simulink model "MCity_cs_withAEBSBlock"  (R2017a)
settings: Solver=ode5  StartTime=0.0  StopTime=3.95  FixedStep=1/200  RelTol=1e-3
PreLoadFcn:
  | check_NUTS_defined;
  | 
  | assignin('base',['model_closed_' bdroot],false);
InitFcn:
  | PreScanExperimentInitFcn(bdroot)
StopFcn:
  | PreScanExperimentStopFcn(bdroot)
model workspace (MAT data in the model file):
  mbox_table : struct (value not decoded)
  model_closed = 0
  sim_status = 0
values from neighbouring files (symbols this model uses):
  d_offset = -18.15    [monocityTestLeftTurn.mat]    (also in simulation_leftTurn_PreScan.m = dl/vl*vh - 43 + R)
undefined symbols (not defined in the file or in its folder): DiscIntNeverNeededParam, warningInitialVelocity, x0
libraries: simulink x78, PreScanSimulinkLibrary x14, simulink_extras x10, PreScanUsefulBlocks x4
(part 2 of 12)

== system MCity_cs_withAEBSBlock/STATE_BMW_Z3_1 ==
  State : Inport  SampleTime=TimeStep
  Acceleration : Subsystem  mask(ToSensorWorld){PortName=Acceleration_BMW_Z3_1, PortIndex=21, PortWidth=3, TimeStep=1/200}
      mask prompts: PortName "Port Name [-]"; PortIndex "Index [-]"; PortWidth "Port Dimensions [-]"; TimeStep "Upload Period [s]"
      mask help: Sends signal(s) from Simulink to the Sensor World
      mask Help:
      | Sends signal(s) from Simulink to the Sensor World.
      | 
      | - Port Name [-]: specifies the name of the output terminal of the Simulink block.
      | - Index [-]: specifies the start position in the output vector sent to the Sensor World
      | - Port dimensions [-]: specifies the width (number of scalars) of the output port
      | - Upload period [s]: specifies the upload period (in seconds) of the port.
      mask Display: port_label('input', 1, PortName)
  Demux : Demux  Outputs=5
  Position : Subsystem  mask(ToSensorWorld){PortName=Position_BMW_Z3_1, PortIndex=15, PortWidth=3, TimeStep=1/200}
      mask prompts: PortName "Port Name [-]"; PortIndex "Index [-]"; PortWidth "Port Dimensions [-]"; TimeStep "Upload Period [s]"
      mask help: Sends signal(s) from Simulink to the Sensor World
      mask Help:
      | Sends signal(s) from Simulink to the Sensor World.
      | 
      | - Port Name [-]: specifies the name of the output terminal of the Simulink block.
      | - Index [-]: specifies the start position in the output vector sent to the Sensor World
      | - Port dimensions [-]: specifies the width (number of scalars) of the output port
      | - Upload period [s]: specifies the upload period (in seconds) of the port.
      mask Display: port_label('input', 1, PortName)
  RPY : Subsystem  mask(ToSensorWorld){PortName=RPY_BMW_Z3_1, PortIndex=24, PortWidth=3, TimeStep=1/200}
      mask prompts: PortName "Port Name [-]"; PortIndex "Index [-]"; PortWidth "Port Dimensions [-]"; TimeStep "Upload Period [s]"
      mask help: Sends signal(s) from Simulink to the Sensor World
      mask Help:
      | Sends signal(s) from Simulink to the Sensor World.
      | 
      | - Port Name [-]: specifies the name of the output terminal of the Simulink block.
      | - Index [-]: specifies the start position in the output vector sent to the Sensor World
      | - Port dimensions [-]: specifies the width (number of scalars) of the output port
      | - Upload period [s]: specifies the upload period (in seconds) of the port.
      mask Display: port_label('input', 1, PortName)
  Velocity : Subsystem  mask(ToSensorWorld){PortName=Velocity_BMW_Z3_1, PortIndex=18, PortWidth=3, TimeStep=1/200}
      mask prompts: PortName "Port Name [-]"; PortIndex "Index [-]"; PortWidth "Port Dimensions [-]"; TimeStep "Upload Period [s]"
      mask help: Sends signal(s) from Simulink to the Sensor World
      mask Help:
      | Sends signal(s) from Simulink to the Sensor World.
      | 
      | - Port Name [-]: specifies the name of the output terminal of the Simulink block.
      | - Index [-]: specifies the start position in the output vector sent to the Sensor World
      | - Port dimensions [-]: specifies the width (number of scalars) of the output port
      | - Upload period [s]: specifies the upload period (in seconds) of the port.
      mask Display: port_label('input', 1, PortName)
  iniBODYAngles wrtVEH [rad] : Constant  Value=[Roll0 Pitch0 0]  SampleTime=TimeStep
  iniVEHAngles wrtGLOB [rad] : Constant  Value=[0 0 Yaw0]  SampleTime=TimeStep
  iniVEHposition wrtGLOB [m] : Constant  Value=[x0 y0+d_offset z0]  SampleTime=TimeStep
  state2FullState : PreScanSimulinkLibrary/state2FullState  SystemSampleTime=-1
  velRPY : Subsystem  mask(ToSensorWorld){PortName=velRPY_BMW_Z3_1, PortIndex=27, PortWidth=3, TimeStep=1/200}
      mask prompts: PortName "Port Name [-]"; PortIndex "Index [-]"; PortWidth "Port Dimensions [-]"; TimeStep "Upload Period [s]"
      mask help: Sends signal(s) from Simulink to the Sensor World
      mask Help:
      | Sends signal(s) from Simulink to the Sensor World.
      | 
      | - Port Name [-]: specifies the name of the output terminal of the Simulink block.
      | - Index [-]: specifies the start position in the output vector sent to the Sensor World
      | - Port dimensions [-]: specifies the width (number of scalars) of the output port
      | - Upload period [s]: specifies the upload period (in seconds) of the port.
      mask Display: port_label('input', 1, PortName)
  wires:
  Demux/5 -> velRPY/1(Y)
  Demux/4 -> RPY/1(Y)
  Demux/3 -> Acceleration/1(Y)
  Demux/2 -> Velocity/1(Y)
  Demux/1 -> Position/1(Y)
  State/1 -> state2FullState/1
  state2FullState/1 -> Demux/1
  iniVEHposition wrtGLOB [m]/1 -> state2FullState/2
  iniBODYAngles wrtVEH [rad]/1 -> state2FullState/3
  iniVEHAngles wrtGLOB [rad]/1 -> state2FullState/4

== system MCity_cs_withAEBSBlock/SetActuators ==
  Bus Creator : BusCreator  Inputs=1
  Data Store Read : DataStoreRead  DataStoreName=SimCoreActuators  SampleTime=TimeStep
  SendActuators : M-S-Function  FunctionName=SendActuatorsBlock  Parameters=TimeStep NrOfActuators
  dummy : Outport
  tag scope: SimCoreInfo=global
  wires:
  Bus Creator/1 -> [SimCoreInfo]  "SimCore"
  SendActuators/2 -> Bus Creator/1  "ComputationTime[s]"
  SendActuators/1 -> dummy/1
  Data Store Read/1 -> SendActuators/1

== system MCity_cs_withAEBSBlock/SimCoreInfo ==
  Bus Selector : BusSelector  OutputSignals=ComputationTime[s]
  Time : Scope
  wires:
  Bus Selector/1 -> Time/1  "<ComputationTime[s]>"
  [SimCoreInfo] -> Bus Selector/1

== system MCity_cs_withAEBSBlock/TrafficLightDoubleUS_1 ==
  Ground_1 : Ground
  "Traffic_Light On/Off " : Subsystem
  VISUCasingLights_1_Mux : Subsystem  Tag=MuxCasingLights  mask(PreScan Mux Block:){}
      settings: DeleteFcn=PreScanBlockDeleteFcn;
  VISUCasingLights_2_Mux : Subsystem  Tag=MuxCasingLights  mask(PreScan Mux Block:){}
      settings: DeleteFcn=PreScanBlockDeleteFcn;
  VISUCasingLights_1_TrafficLightDoubleUS_1 : Outport  Tag=VisuCasingLights_1Outport  SampleTime=1/200
  VISUCasingLights_2_TrafficLightDoubleUS_1 : Outport  Tag=VisuCasingLights_2Outport  Port=2  SampleTime=1/200
  wires:
  VISUCasingLights_2_Mux/1(CasingLights) -> VISUCasingLights_2_TrafficLightDoubleUS_1/1
  VISUCasingLights_1_Mux/1(CasingLights) -> VISUCasingLights_1_TrafficLightDoubleUS_1/1
  "Traffic_Light On/Off "/3(Green) -> VISUCasingLights_1_Mux/3(Green [-]), VISUCasingLights_2_Mux/3(Green [-])
  "Traffic_Light On/Off "/2(Orange) -> VISUCasingLights_1_Mux/2(Orange [-]), VISUCasingLights_2_Mux/2(Orange [-])
  "Traffic_Light On/Off "/1(Red) -> VISUCasingLights_1_Mux/1(Red [-]), VISUCasingLights_2_Mux/1(Red [-])

== system MCity_cs_withAEBSBlock/TrafficLightDoubleUS_10 ==
  Perpendicular : Subsystem
  VISUCasingLights_1_Mux : Subsystem  Tag=MuxCasingLights  mask(PreScan Mux Block:){}
      settings: DeleteFcn=PreScanBlockDeleteFcn;
  VISUCasingLights_2_Mux : Subsystem  Tag=MuxCasingLights  mask(PreScan Mux Block:){}
      settings: DeleteFcn=PreScanBlockDeleteFcn;
  VISUCasingLights_1_TrafficLightDoubleUS_10 : Outport  Tag=VisuCasingLights_1Outport  SampleTime=1/200
  VISUCasingLights_2_TrafficLightDoubleUS_10 : Outport  Tag=VisuCasingLights_2Outport  Port=2  SampleTime=1/200
  wires:
  VISUCasingLights_2_Mux/1(CasingLights) -> VISUCasingLights_2_TrafficLightDoubleUS_10/1
  VISUCasingLights_1_Mux/1(CasingLights) -> VISUCasingLights_1_TrafficLightDoubleUS_10/1
  Perpendicular/3(Green) -> VISUCasingLights_1_Mux/3(Green [-]), VISUCasingLights_2_Mux/3(Green [-])
  Perpendicular/2(Orange) -> VISUCasingLights_1_Mux/2(Orange [-]), VISUCasingLights_2_Mux/2(Orange [-])
  Perpendicular/1(Red) -> VISUCasingLights_1_Mux/1(Red [-]), VISUCasingLights_2_Mux/1(Red [-])

== system MCity_cs_withAEBSBlock/TrafficLightDoubleUS_2 ==
  Ground_1 : Ground
  "Traffic_Light On/Off " : Subsystem
  VISUCasingLights_1_Mux : Subsystem  Tag=MuxCasingLights  mask(PreScan Mux Block:){}
      settings: DeleteFcn=PreScanBlockDeleteFcn;
  VISUCasingLights_2_Mux : Subsystem  Tag=MuxCasingLights  mask(PreScan Mux Block:){}
      settings: DeleteFcn=PreScanBlockDeleteFcn;
  VISUCasingLights_1_TrafficLightDoubleUS_2 : Outport  Tag=VisuCasingLights_1Outport  SampleTime=1/200
  VISUCasingLights_2_TrafficLightDoubleUS_2 : Outport  Tag=VisuCasingLights_2Outport  Port=2  SampleTime=1/200
  wires:
  VISUCasingLights_2_Mux/1(CasingLights) -> VISUCasingLights_2_TrafficLightDoubleUS_2/1
  VISUCasingLights_1_Mux/1(CasingLights) -> VISUCasingLights_1_TrafficLightDoubleUS_2/1
  "Traffic_Light On/Off "/3(Green) -> VISUCasingLights_1_Mux/3(Green [-]), VISUCasingLights_2_Mux/3(Green [-])
  "Traffic_Light On/Off "/2(Orange) -> VISUCasingLights_1_Mux/2(Orange [-]), VISUCasingLights_2_Mux/2(Orange [-])
  "Traffic_Light On/Off "/1(Red) -> VISUCasingLights_1_Mux/1(Red [-]), VISUCasingLights_2_Mux/1(Red [-])

== system MCity_cs_withAEBSBlock/TrafficLightDoubleUS_3 ==
  Perpendicular : Subsystem
  VISUCasingLights_1_Mux : Subsystem  Tag=MuxCasingLights  mask(PreScan Mux Block:){}
      settings: DeleteFcn=PreScanBlockDeleteFcn;
  VISUCasingLights_2_Mux : Subsystem  Tag=MuxCasingLights  mask(PreScan Mux Block:){}
      settings: DeleteFcn=PreScanBlockDeleteFcn;
  VISUCasingLights_1_TrafficLightDoubleUS_3 : Outport  Tag=VisuCasingLights_1Outport  SampleTime=1/200
  VISUCasingLights_2_TrafficLightDoubleUS_3 : Outport  Tag=VisuCasingLights_2Outport  Port=2  SampleTime=1/200
  wires:
  VISUCasingLights_2_Mux/1(CasingLights) -> VISUCasingLights_2_TrafficLightDoubleUS_3/1
  VISUCasingLights_1_Mux/1(CasingLights) -> VISUCasingLights_1_TrafficLightDoubleUS_3/1
  Perpendicular/3(Green) -> VISUCasingLights_1_Mux/3(Green [-]), VISUCasingLights_2_Mux/3(Green [-])
  Perpendicular/2(Orange) -> VISUCasingLights_1_Mux/2(Orange [-]), VISUCasingLights_2_Mux/2(Orange [-])
  Perpendicular/1(Red) -> VISUCasingLights_1_Mux/1(Red [-]), VISUCasingLights_2_Mux/1(Red [-])

== system MCity_cs_withAEBSBlock/TrafficLightDoubleUS_4 ==
  Perpendicular : Subsystem
  VISUCasingLights_1_Mux : Subsystem  Tag=MuxCasingLights  mask(PreScan Mux Block:){}
      settings: DeleteFcn=PreScanBlockDeleteFcn;
  VISUCasingLights_2_Mux : Subsystem  Tag=MuxCasingLights  mask(PreScan Mux Block:){}
      settings: DeleteFcn=PreScanBlockDeleteFcn;
  VISUCasingLights_1_TrafficLightDoubleUS_4 : Outport  Tag=VisuCasingLights_1Outport  SampleTime=1/200
  VISUCasingLights_2_TrafficLightDoubleUS_4 : Outport  Tag=VisuCasingLights_2Outport  Port=2  SampleTime=1/200
  wires:
  VISUCasingLights_2_Mux/1(CasingLights) -> VISUCasingLights_2_TrafficLightDoubleUS_4/1
  VISUCasingLights_1_Mux/1(CasingLights) -> VISUCasingLights_1_TrafficLightDoubleUS_4/1
  Perpendicular/3(Green) -> VISUCasingLights_1_Mux/3(Green [-]), VISUCasingLights_2_Mux/3(Green [-])
  Perpendicular/2(Orange) -> VISUCasingLights_1_Mux/2(Orange [-]), VISUCasingLights_2_Mux/2(Orange [-])
  Perpendicular/1(Red) -> VISUCasingLights_1_Mux/1(Red [-]), VISUCasingLights_2_Mux/1(Red [-])

== system MCity_cs_withAEBSBlock/TrafficLightDoubleUS_5 ==
  Ground_{1..6} (6 alike) : Ground
  Terminator_{1..5} (5 alike) : Terminator
  "Traffic_Light On/Off " : Subsystem
  VISUCasingLights_1_Mux : Subsystem  Tag=MuxCasingLights  mask(PreScan Mux Block:){}
      settings: DeleteFcn=PreScanBlockDeleteFcn;
  VISUCasingLights_2_Mux : Subsystem  Tag=MuxCasingLights  mask(PreScan Mux Block:){}
      settings: DeleteFcn=PreScanBlockDeleteFcn;
  VISUCasingLights_1_TrafficLightDoubleUS_5 : Outport  Tag=VisuCasingLights_1Outport  SampleTime=1/200
  VISUCasingLights_2_TrafficLightDoubleUS_5 : Outport  Tag=VisuCasingLights_2Outport  Port=2  SampleTime=1/200
  wires:
  VISUCasingLights_2_Mux/1(CasingLights) -> VISUCasingLights_2_TrafficLightDoubleUS_5/1
  VISUCasingLights_1_Mux/1(CasingLights) -> VISUCasingLights_1_TrafficLightDoubleUS_5/1
  "Traffic_Light On/Off "/3(Green) -> VISUCasingLights_2_Mux/3(Green [-]), VISUCasingLights_1_Mux/3(Green [-])
  "Traffic_Light On/Off "/2(Orange) -> VISUCasingLights_2_Mux/2(Orange [-]), VISUCasingLights_1_Mux/2(Orange [-])
  "Traffic_Light On/Off "/1(Red) -> VISUCasingLights_2_Mux/1(Red [-]), VISUCasingLights_1_Mux/1(Red [-])
  Ground_1/1 -> Terminator_1/1
  Ground_2/1 -> Terminator_2/1
  Ground_3/1 -> Terminator_3/1
  Ground_4/1 -> Terminator_4/1
  Ground_5/1 -> Terminator_5/1

== system MCity_cs_withAEBSBlock/TrafficLightDoubleUS_6 ==
  Ground_1 : Ground
  "Traffic_Light On/Off " : Subsystem
  VISUCasingLights_1_Mux : Subsystem  Tag=MuxCasingLights  mask(PreScan Mux Block:){}
      settings: DeleteFcn=PreScanBlockDeleteFcn;
  VISUCasingLights_2_Mux : Subsystem  Tag=MuxCasingLights  mask(PreScan Mux Block:){}
      settings: DeleteFcn=PreScanBlockDeleteFcn;
  VISUCasingLights_1_TrafficLightDoubleUS_6 : Outport  Tag=VisuCasingLights_1Outport  SampleTime=1/200
  VISUCasingLights_2_TrafficLightDoubleUS_6 : Outport  Tag=VisuCasingLights_2Outport  Port=2  SampleTime=1/200
  wires:
  VISUCasingLights_2_Mux/1(CasingLights) -> VISUCasingLights_2_TrafficLightDoubleUS_6/1
  VISUCasingLights_1_Mux/1(CasingLights) -> VISUCasingLights_1_TrafficLightDoubleUS_6/1
  "Traffic_Light On/Off "/3(Green) -> VISUCasingLights_1_Mux/3(Green [-]), VISUCasingLights_2_Mux/3(Green [-])
  "Traffic_Light On/Off "/2(Orange) -> VISUCasingLights_1_Mux/2(Orange [-]), VISUCasingLights_2_Mux/2(Orange [-])
  "Traffic_Light On/Off "/1(Red) -> VISUCasingLights_1_Mux/1(Red [-]), VISUCasingLights_2_Mux/1(Red [-])

== system MCity_cs_withAEBSBlock/TrafficLightDoubleUS_7 ==
  Ground_1 : Ground
  "Traffic_Light On/Off " : Subsystem
  VISUCasingLights_1_Mux : Subsystem  Tag=MuxCasingLights  mask(PreScan Mux Block:){}
      settings: DeleteFcn=PreScanBlockDeleteFcn;
  VISUCasingLights_2_Mux : Subsystem  Tag=MuxCasingLights  mask(PreScan Mux Block:){}
      settings: DeleteFcn=PreScanBlockDeleteFcn;
  VISUCasingLights_1_TrafficLightDoubleUS_7 : Outport  Tag=VisuCasingLights_1Outport  SampleTime=1/200
  VISUCasingLights_2_TrafficLightDoubleUS_7 : Outport  Tag=VisuCasingLights_2Outport  Port=2  SampleTime=1/200
  wires:
  VISUCasingLights_2_Mux/1(CasingLights) -> VISUCasingLights_2_TrafficLightDoubleUS_7/1
  VISUCasingLights_1_Mux/1(CasingLights) -> VISUCasingLights_1_TrafficLightDoubleUS_7/1
  "Traffic_Light On/Off "/3(Green) -> VISUCasingLights_1_Mux/3(Green [-]), VISUCasingLights_2_Mux/3(Green [-])
  "Traffic_Light On/Off "/2(Orange) -> VISUCasingLights_1_Mux/2(Orange [-]), VISUCasingLights_2_Mux/2(Orange [-])
  "Traffic_Light On/Off "/1(Red) -> VISUCasingLights_1_Mux/1(Red [-]), VISUCasingLights_2_Mux/1(Red [-])

== system MCity_cs_withAEBSBlock/TrafficLightDoubleUS_8 ==
  Ground_{1..7} (7 alike) : Ground
  Terminator_{1..6} (6 alike) : Terminator
  "Traffic_Light On/Off " : Subsystem
  VISUCasingLights_1_Mux : Subsystem  Tag=MuxCasingLights  mask(PreScan Mux Block:){}
      settings: DeleteFcn=PreScanBlockDeleteFcn;
  VISUCasingLights_2_Mux : Subsystem  Tag=MuxCasingLights  mask(PreScan Mux Block:){}
      settings: DeleteFcn=PreScanBlockDeleteFcn;
  VISUCasingLights_1_TrafficLightDoubleUS_8 : Outport  Tag=VisuCasingLights_1Outport  SampleTime=1/200
  VISUCasingLights_2_TrafficLightDoubleUS_8 : Outport  Tag=VisuCasingLights_2Outport  Port=2  SampleTime=1/200
  wires:
  VISUCasingLights_2_Mux/1(CasingLights) -> VISUCasingLights_2_TrafficLightDoubleUS_8/1
  VISUCasingLights_1_Mux/1(CasingLights) -> VISUCasingLights_1_TrafficLightDoubleUS_8/1
  "Traffic_Light On/Off "/3(Green) -> VISUCasingLights_1_Mux/3(Green [-]), VISUCasingLights_2_Mux/3(Green [-])
  "Traffic_Light On/Off "/2(Orange) -> VISUCasingLights_1_Mux/2(Orange [-]), VISUCasingLights_2_Mux/2(Orange [-])
  "Traffic_Light On/Off "/1(Red) -> VISUCasingLights_1_Mux/1(Red [-]), VISUCasingLights_2_Mux/1(Red [-])
  Ground_1/1 -> Terminator_1/1
  Ground_2/1 -> Terminator_2/1
  Ground_3/1 -> Terminator_3/1
  Ground_4/1 -> Terminator_4/1
  Ground_5/1 -> Terminator_5/1
  Ground_6/1 -> Terminator_6/1

== system MCity_cs_withAEBSBlock/TrafficLightDoubleUS_9 ==
  Ground_1 : Ground
  "Traffic_Light On/Off " : Subsystem
  VISUCasingLights_1_Mux : Subsystem  Tag=MuxCasingLights  mask(PreScan Mux Block:){}
      settings: DeleteFcn=PreScanBlockDeleteFcn;
  VISUCasingLights_2_Mux : Subsystem  Tag=MuxCasingLights  mask(PreScan Mux Block:){}
      settings: DeleteFcn=PreScanBlockDeleteFcn;
  VISUCasingLights_1_TrafficLightDoubleUS_9 : Outport  Tag=VisuCasingLights_1Outport  SampleTime=1/200
  VISUCasingLights_2_TrafficLightDoubleUS_9 : Outport  Tag=VisuCasingLights_2Outport  Port=2  SampleTime=1/200
  wires:
  VISUCasingLights_2_Mux/1(CasingLights) -> VISUCasingLights_2_TrafficLightDoubleUS_9/1
  VISUCasingLights_1_Mux/1(CasingLights) -> VISUCasingLights_1_TrafficLightDoubleUS_9/1
  "Traffic_Light On/Off "/3(Green) -> VISUCasingLights_1_Mux/3(Green [-]), VISUCasingLights_2_Mux/3(Green [-])
  "Traffic_Light On/Off "/2(Orange) -> VISUCasingLights_1_Mux/2(Orange [-]), VISUCasingLights_2_Mux/2(Orange [-])
  "Traffic_Light On/Off "/1(Red) -> VISUCasingLights_1_Mux/1(Red [-]), VISUCasingLights_2_Mux/1(Red [-])

== system MCity_cs_withAEBSBlock/TrafficLightSingleUS_1 ==
  Perpendicular : Subsystem
  VISUCasingLights_Mux : Subsystem  Tag=MuxCasingLights  mask(PreScan Mux Block:){}
      settings: DeleteFcn=PreScanBlockDeleteFcn;
  VISUCasingLights_TrafficLightSingleUS_1 : Outport  Tag=VisuCasingLightsOutport  SampleTime=1/200
  wires:
  VISUCasingLights_Mux/1(CasingLights) -> VISUCasingLights_TrafficLightSingleUS_1/1
  Perpendicular/3(Green) -> VISUCasingLights_Mux/3(Green [-])
  Perpendicular/2(Orange) -> VISUCasingLights_Mux/2(Orange [-])
  Perpendicular/1(Red) -> VISUCasingLights_Mux/1(Red [-])

== system MCity_cs_withAEBSBlock/TrafficLightSingleUS_2 ==
  Traffic_Light_Perpendicular : Subsystem
  VISUCasingLights_Mux : Subsystem  Tag=MuxCasingLights  mask(PreScan Mux Block:){}
      settings: DeleteFcn=PreScanBlockDeleteFcn;
  VISUCasingLights_TrafficLightSingleUS_2 : Outport  Tag=VisuCasingLightsOutport  SampleTime=1/200
  wires:
  VISUCasingLights_Mux/1(CasingLights) -> VISUCasingLights_TrafficLightSingleUS_2/1
  Traffic_Light_Perpendicular/3(Green) -> VISUCasingLights_Mux/3(Green [-])
  Traffic_Light_Perpendicular/2(Orange) -> VISUCasingLights_Mux/2(Orange [-])
  Traffic_Light_Perpendicular/1(Red) -> VISUCasingLights_Mux/1(Red [-])

== system MCity_cs_withAEBSBlock/VISUCasingLights_1_TrafficLightDoubleUS_1 ==
  CasingLights : Inport
  Demux4 : Demux  Outputs=3
  Saturation1 : Saturate  UpperLimit=1  LowerLimit=0
  Saturation2 : Saturate  UpperLimit=1  LowerLimit=0
  Saturation3 : Saturate  UpperLimit=1  LowerLimit=0
  conv_Green : Subsystem
  conv_Orange : Subsystem
  conv_Red : Subsystem
  visu_CasingGreen : Subsystem  mask(ToSensorWorld){PortName=visu_LightCasingGreen_1, PortIndex=30, PortWidth=16, TimeStep=1/200}
      mask prompts: PortName "Port Name [-]"; PortIndex "Index [-]"; PortWidth "Port Dimensions [-]"; TimeStep "Upload Period [s]"
      mask help: Sends signal(s) from Simulink to the Sensor World
      mask Help:
      | Sends signal(s) from Simulink to the Sensor World.
      | 
      | - Port Name [-]: specifies the name of the output terminal of the Simulink block.
      | - Index [-]: specifies the start position in the output vector sent to the Sensor World
      | - Port dimensions [-]: specifies the width (number of scalars) of the output port
      | - Upload period [s]: specifies the upload period (in seconds) of the port.
      mask Display: port_label('input', 1, PortName)
  visu_CasingOrange : Subsystem  mask(ToSensorWorld){PortName=visu_LightCasingOrange_1, PortIndex=46, PortWidth=16, TimeStep=1/200}
      mask prompts: PortName "Port Name [-]"; PortIndex "Index [-]"; PortWidth "Port Dimensions [-]"; TimeStep "Upload Period [s]"
      mask help: Sends signal(s) from Simulink to the Sensor World
      mask Help:
      | Sends signal(s) from Simulink to the Sensor World.
      | 
      | - Port Name [-]: specifies the name of the output terminal of the Simulink block.
      | - Index [-]: specifies the start position in the output vector sent to the Sensor World
      | - Port dimensions [-]: specifies the width (number of scalars) of the output port
      | - Upload period [s]: specifies the upload period (in seconds) of the port.
      mask Display: port_label('input', 1, PortName)
  visu_CasingRed : Subsystem  mask(ToSensorWorld){PortName=visu_LightCasingRed_1, PortIndex=62, PortWidth=16, TimeStep=1/200}
      mask prompts: PortName "Port Name [-]"; PortIndex "Index [-]"; PortWidth "Port Dimensions [-]"; TimeStep "Upload Period [s]"
      mask help: Sends signal(s) from Simulink to the Sensor World
      mask Help:
      | Sends signal(s) from Simulink to the Sensor World.
      | 
      | - Port Name [-]: specifies the name of the output terminal of the Simulink block.
      | - Index [-]: specifies the start position in the output vector sent to the Sensor World
      | - Port dimensions [-]: specifies the width (number of scalars) of the output port
      | - Upload period [s]: specifies the upload period (in seconds) of the port.
      mask Display: port_label('input', 1, PortName)
  wires:
  CasingLights/1 -> Demux4/1
  Demux4/3 -> Saturation3/1
  Demux4/2 -> Saturation2/1
  Demux4/1 -> Saturation1/1
  Saturation1/1 -> conv_Red/1(on_off)
  Saturation2/1 -> conv_Orange/1(on_off)
  Saturation3/1 -> conv_Green/1(on_off)
  conv_Red/1(RGBcolor) -> visu_CasingRed/1(Y)
  conv_Orange/1(RGBcolor) -> visu_CasingOrange/1(Y)
  conv_Green/1(RGBcolor) -> visu_CasingGreen/1(Y)

== system MCity_cs_withAEBSBlock/VISUCasingLights_1_TrafficLightDoubleUS_10 ==
  CasingLights : Inport
  Demux4 : Demux  Outputs=3
  Saturation1 : Saturate  UpperLimit=1  LowerLimit=0
  Saturation2 : Saturate  UpperLimit=1  LowerLimit=0
  Saturation3 : Saturate  UpperLimit=1  LowerLimit=0
  conv_Green : Subsystem
  conv_Orange : Subsystem
  conv_Red : Subsystem
  visu_CasingGreen : Subsystem  mask(ToSensorWorld){PortName=visu_LightCasingGreen_1, PortIndex=798, PortWidth=16, TimeStep=1/200}
      mask prompts: PortName "Port Name [-]"; PortIndex "Index [-]"; PortWidth "Port Dimensions [-]"; TimeStep "Upload Period [s]"
      mask help: Sends signal(s) from Simulink to the Sensor World
      mask Help:
      | Sends signal(s) from Simulink to the Sensor World.
      | 
      | - Port Name [-]: specifies the name of the output terminal of the Simulink block.
      | - Index [-]: specifies the start position in the output vector sent to the Sensor World
      | - Port dimensions [-]: specifies the width (number of scalars) of the output port
      | - Upload period [s]: specifies the upload period (in seconds) of the port.
      mask Display: port_label('input', 1, PortName)
  visu_CasingOrange : Subsystem  mask(ToSensorWorld){PortName=visu_LightCasingOrange_1, PortIndex=814, PortWidth=16, TimeStep=1/200}
      mask prompts: PortName "Port Name [-]"; PortIndex "Index [-]"; PortWidth "Port Dimensions [-]"; TimeStep "Upload Period [s]"
      mask help: Sends signal(s) from Simulink to the Sensor World
      mask Help:
      | Sends signal(s) from Simulink to the Sensor World.
      | 
      | - Port Name [-]: specifies the name of the output terminal of the Simulink block.
      | - Index [-]: specifies the start position in the output vector sent to the Sensor World
      | - Port dimensions [-]: specifies the width (number of scalars) of the output port
      | - Upload period [s]: specifies the upload period (in seconds) of the port.
      mask Display: port_label('input', 1, PortName)
  visu_CasingRed : Subsystem  mask(ToSensorWorld){PortName=visu_LightCasingRed_1, PortIndex=830, PortWidth=16, TimeStep=1/200}
      mask prompts: PortName "Port Name [-]"; PortIndex "Index [-]"; PortWidth "Port Dimensions [-]"; TimeStep "Upload Period [s]"
      mask help: Sends signal(s) from Simulink to the Sensor World
      mask Help:
      | Sends signal(s) from Simulink to the Sensor World.
      | 
      | - Port Name [-]: specifies the name of the output terminal of the Simulink block.
      | - Index [-]: specifies the start position in the output vector sent to the Sensor World
      | - Port dimensions [-]: specifies the width (number of scalars) of the output port
      | - Upload period [s]: specifies the upload period (in seconds) of the port.
      mask Display: port_label('input', 1, PortName)
  wires:
  CasingLights/1 -> Demux4/1
  Demux4/3 -> Saturation3/1
  Demux4/2 -> Saturation2/1
  Demux4/1 -> Saturation1/1
  Saturation1/1 -> conv_Red/1(on_off)
  Saturation2/1 -> conv_Orange/1(on_off)
  Saturation3/1 -> conv_Green/1(on_off)
  conv_Red/1(RGBcolor) -> visu_CasingRed/1(Y)
  conv_Orange/1(RGBcolor) -> visu_CasingOrange/1(Y)
  conv_Green/1(RGBcolor) -> visu_CasingGreen/1(Y)

== system MCity_cs_withAEBSBlock/VISUCasingLights_1_TrafficLightDoubleUS_2 ==
  CasingLights : Inport
  Demux4 : Demux  Outputs=3
  Saturation1 : Saturate  UpperLimit=1  LowerLimit=0
  Saturation2 : Saturate  UpperLimit=1  LowerLimit=0
  Saturation3 : Saturate  UpperLimit=1  LowerLimit=0
  conv_Green : Subsystem
  conv_Orange : Subsystem
  conv_Red : Subsystem
  visu_CasingGreen : Subsystem  mask(ToSensorWorld){PortName=visu_LightCasingGreen_1, PortIndex=126, PortWidth=16, TimeStep=1/200}
      mask prompts: PortName "Port Name [-]"; PortIndex "Index [-]"; PortWidth "Port Dimensions [-]"; TimeStep "Upload Period [s]"
      mask help: Sends signal(s) from Simulink to the Sensor World
      mask Help:
      | Sends signal(s) from Simulink to the Sensor World.
      | 
      | - Port Name [-]: specifies the name of the output terminal of the Simulink block.
      | - Index [-]: specifies the start position in the output vector sent to the Sensor World
      | - Port dimensions [-]: specifies the width (number of scalars) of the output port
      | - Upload period [s]: specifies the upload period (in seconds) of the port.
      mask Display: port_label('input', 1, PortName)
  visu_CasingOrange : Subsystem  mask(ToSensorWorld){PortName=visu_LightCasingOrange_1, PortIndex=142, PortWidth=16, TimeStep=1/200}
      mask prompts: PortName "Port Name [-]"; PortIndex "Index [-]"; PortWidth "Port Dimensions [-]"; TimeStep "Upload Period [s]"
      mask help: Sends signal(s) from Simulink to the Sensor World
      mask Help:
      | Sends signal(s) from Simulink to the Sensor World.
      | 
      | - Port Name [-]: specifies the name of the output terminal of the Simulink block.
      | - Index [-]: specifies the start position in the output vector sent to the Sensor World
      | - Port dimensions [-]: specifies the width (number of scalars) of the output port
      | - Upload period [s]: specifies the upload period (in seconds) of the port.
      mask Display: port_label('input', 1, PortName)
  visu_CasingRed : Subsystem  mask(ToSensorWorld){PortName=visu_LightCasingRed_1, PortIndex=158, PortWidth=16, TimeStep=1/200}
      mask prompts: PortName "Port Name [-]"; PortIndex "Index [-]"; PortWidth "Port Dimensions [-]"; TimeStep "Upload Period [s]"
      mask help: Sends signal(s) from Simulink to the Sensor World
      mask Help:
      | Sends signal(s) from Simulink to the Sensor World.
      | 
      | - Port Name [-]: specifies the name of the output terminal of the Simulink block.
      | - Index [-]: specifies the start position in the output vector sent to the Sensor World
      | - Port dimensions [-]: specifies the width (number of scalars) of the output port
      | - Upload period [s]: specifies the upload period (in seconds) of the port.
      mask Display: port_label('input', 1, PortName)
  wires:
  CasingLights/1 -> Demux4/1
  Demux4/3 -> Saturation3/1
  Demux4/2 -> Saturation2/1
  Demux4/1 -> Saturation1/1
  Saturation1/1 -> conv_Red/1(on_off)
  Saturation2/1 -> conv_Orange/1(on_off)
  Saturation3/1 -> conv_Green/1(on_off)
  conv_Red/1(RGBcolor) -> visu_CasingRed/1(Y)
  conv_Orange/1(RGBcolor) -> visu_CasingOrange/1(Y)
  conv_Green/1(RGBcolor) -> visu_CasingGreen/1(Y)

== system MCity_cs_withAEBSBlock/VISUCasingLights_1_TrafficLightDoubleUS_3 ==
  CasingLights : Inport
  Demux4 : Demux  Outputs=3
  Saturation1 : Saturate  UpperLimit=1  LowerLimit=0
  Saturation2 : Saturate  UpperLimit=1  LowerLimit=0
  Saturation3 : Saturate  UpperLimit=1  LowerLimit=0
  conv_Green : Subsystem
  conv_Orange : Subsystem
  conv_Red : Subsystem
  visu_CasingGreen : Subsystem  mask(ToSensorWorld){PortName=visu_LightCasingGreen_1, PortIndex=222, PortWidth=16, TimeStep=1/200}
      mask prompts: PortName "Port Name [-]"; PortIndex "Index [-]"; PortWidth "Port Dimensions [-]"; TimeStep "Upload Period [s]"
      mask help: Sends signal(s) from Simulink to the Sensor World
      mask Help:
      | Sends signal(s) from Simulink to the Sensor World.
      | 
      | - Port Name [-]: specifies the name of the output terminal of the Simulink block.
      | - Index [-]: specifies the start position in the output vector sent to the Sensor World
      | - Port dimensions [-]: specifies the width (number of scalars) of the output port
      | - Upload period [s]: specifies the upload period (in seconds) of the port.
      mask Display: port_label('input', 1, PortName)
  visu_CasingOrange : Subsystem  mask(ToSensorWorld){PortName=visu_LightCasingOrange_1, PortIndex=238, PortWidth=16, TimeStep=1/200}
      mask prompts: PortName "Port Name [-]"; PortIndex "Index [-]"; PortWidth "Port Dimensions [-]"; TimeStep "Upload Period [s]"
      mask help: Sends signal(s) from Simulink to the Sensor World
      mask Help:
      | Sends signal(s) from Simulink to the Sensor World.
      | 
      | - Port Name [-]: specifies the name of the output terminal of the Simulink block.
      | - Index [-]: specifies the start position in the output vector sent to the Sensor World
      | - Port dimensions [-]: specifies the width (number of scalars) of the output port
      | - Upload period [s]: specifies the upload period (in seconds) of the port.
      mask Display: port_label('input', 1, PortName)
  visu_CasingRed : Subsystem  mask(ToSensorWorld){PortName=visu_LightCasingRed_1, PortIndex=254, PortWidth=16, TimeStep=1/200}
      mask prompts: PortName "Port Name [-]"; PortIndex "Index [-]"; PortWidth "Port Dimensions [-]"; TimeStep "Upload Period [s]"
      mask help: Sends signal(s) from Simulink to the Sensor World
      mask Help:
      | Sends signal(s) from Simulink to the Sensor World.
      | 
      | - Port Name [-]: specifies the name of the output terminal of the Simulink block.
      | - Index [-]: specifies the start position in the output vector sent to the Sensor World
      | - Port dimensions [-]: specifies the width (number of scalars) of the output port
      | - Upload period [s]: specifies the upload period (in seconds) of the port.
      mask Display: port_label('input', 1, PortName)
  wires:
  CasingLights/1 -> Demux4/1
  Demux4/3 -> Saturation3/1
  Demux4/2 -> Saturation2/1
  Demux4/1 -> Saturation1/1
  Saturation1/1 -> conv_Red/1(on_off)
  Saturation2/1 -> conv_Orange/1(on_off)
  Saturation3/1 -> conv_Green/1(on_off)
  conv_Red/1(RGBcolor) -> visu_CasingRed/1(Y)
  conv_Orange/1(RGBcolor) -> visu_CasingOrange/1(Y)
  conv_Green/1(RGBcolor) -> visu_CasingGreen/1(Y)

== system MCity_cs_withAEBSBlock/VISUCasingLights_1_TrafficLightDoubleUS_4 ==
  CasingLights : Inport
  Demux4 : Demux  Outputs=3
  Saturation1 : Saturate  UpperLimit=1  LowerLimit=0
  Saturation2 : Saturate  UpperLimit=1  LowerLimit=0
  Saturation3 : Saturate  UpperLimit=1  LowerLimit=0
  conv_Green : Subsystem
  conv_Orange : Subsystem
  conv_Red : Subsystem
  visu_CasingGreen : Subsystem  mask(ToSensorWorld){PortName=visu_LightCasingGreen_1, PortIndex=318, PortWidth=16, TimeStep=1/200}
      mask prompts: PortName "Port Name [-]"; PortIndex "Index [-]"; PortWidth "Port Dimensions [-]"; TimeStep "Upload Period [s]"
      mask help: Sends signal(s) from Simulink to the Sensor World
      mask Help:
      | Sends signal(s) from Simulink to the Sensor World.
      | 
      | - Port Name [-]: specifies the name of the output terminal of the Simulink block.
      | - Index [-]: specifies the start position in the output vector sent to the Sensor World
      | - Port dimensions [-]: specifies the width (number of scalars) of the output port
      | - Upload period [s]: specifies the upload period (in seconds) of the port.
      mask Display: port_label('input', 1, PortName)
  visu_CasingOrange : Subsystem  mask(ToSensorWorld){PortName=visu_LightCasingOrange_1, PortIndex=334, PortWidth=16, TimeStep=1/200}
      mask prompts: PortName "Port Name [-]"; PortIndex "Index [-]"; PortWidth "Port Dimensions [-]"; TimeStep "Upload Period [s]"
      mask help: Sends signal(s) from Simulink to the Sensor World
      mask Help:
      | Sends signal(s) from Simulink to the Sensor World.
      | 
      | - Port Name [-]: specifies the name of the output terminal of the Simulink block.
      | - Index [-]: specifies the start position in the output vector sent to the Sensor World
      | - Port dimensions [-]: specifies the width (number of scalars) of the output port
      | - Upload period [s]: specifies the upload period (in seconds) of the port.
      mask Display: port_label('input', 1, PortName)
  visu_CasingRed : Subsystem  mask(ToSensorWorld){PortName=visu_LightCasingRed_1, PortIndex=350, PortWidth=16, TimeStep=1/200}
      mask prompts: PortName "Port Name [-]"; PortIndex "Index [-]"; PortWidth "Port Dimensions [-]"; TimeStep "Upload Period [s]"
      mask help: Sends signal(s) from Simulink to the Sensor World
      mask Help:
      | Sends signal(s) from Simulink to the Sensor World.
      | 
      | - Port Name [-]: specifies the name of the output terminal of the Simulink block.
      | - Index [-]: specifies the start position in the output vector sent to the Sensor World
      | - Port dimensions [-]: specifies the width (number of scalars) of the output port
      | - Upload period [s]: specifies the upload period (in seconds) of the port.
      mask Display: port_label('input', 1, PortName)
  wires:
  CasingLights/1 -> Demux4/1
  Demux4/3 -> Saturation3/1
  Demux4/2 -> Saturation2/1
  Demux4/1 -> Saturation1/1
  Saturation1/1 -> conv_Red/1(on_off)
  Saturation2/1 -> conv_Orange/1(on_off)
  Saturation3/1 -> conv_Green/1(on_off)
  conv_Red/1(RGBcolor) -> visu_CasingRed/1(Y)
  conv_Orange/1(RGBcolor) -> visu_CasingOrange/1(Y)
  conv_Green/1(RGBcolor) -> visu_CasingGreen/1(Y)

== system MCity_cs_withAEBSBlock/VISUCasingLights_1_TrafficLightDoubleUS_5 ==
  CasingLights : Inport
  Demux4 : Demux  Outputs=3
  Saturation1 : Saturate  UpperLimit=1  LowerLimit=0
  Saturation2 : Saturate  UpperLimit=1  LowerLimit=0
  Saturation3 : Saturate  UpperLimit=1  LowerLimit=0
  conv_Green : Subsystem
  conv_Orange : Subsystem
  conv_Red : Subsystem
  visu_CasingGreen : Subsystem  mask(ToSensorWorld){PortName=visu_LightCasingGreen_1, PortIndex=894, PortWidth=16, TimeStep=1/200}
      mask prompts: PortName "Port Name [-]"; PortIndex "Index [-]"; PortWidth "Port Dimensions [-]"; TimeStep "Upload Period [s]"
      mask help: Sends signal(s) from Simulink to the Sensor World
      mask Help:
      | Sends signal(s) from Simulink to the Sensor World.
      | 
      | - Port Name [-]: specifies the name of the output terminal of the Simulink block.
      | - Index [-]: specifies the start position in the output vector sent to the Sensor World
      | - Port dimensions [-]: specifies the width (number of scalars) of the output port
      | - Upload period [s]: specifies the upload period (in seconds) of the port.
      mask Display: port_label('input', 1, PortName)
  visu_CasingOrange : Subsystem  mask(ToSensorWorld){PortName=visu_LightCasingOrange_1, PortIndex=910, PortWidth=16, TimeStep=1/200}
      mask prompts: PortName "Port Name [-]"; PortIndex "Index [-]"; PortWidth "Port Dimensions [-]"; TimeStep "Upload Period [s]"
      mask help: Sends signal(s) from Simulink to the Sensor World
      mask Help:
      | Sends signal(s) from Simulink to the Sensor World.
      | 
      | - Port Name [-]: specifies the name of the output terminal of the Simulink block.
      | - Index [-]: specifies the start position in the output vector sent to the Sensor World
      | - Port dimensions [-]: specifies the width (number of scalars) of the output port
      | - Upload period [s]: specifies the upload period (in seconds) of the port.
      mask Display: port_label('input', 1, PortName)
  visu_CasingRed : Subsystem  mask(ToSensorWorld){PortName=visu_LightCasingRed_1, PortIndex=926, PortWidth=16, TimeStep=1/200}
      mask prompts: PortName "Port Name [-]"; PortIndex "Index [-]"; PortWidth "Port Dimensions [-]"; TimeStep "Upload Period [s]"
      mask help: Sends signal(s) from Simulink to the Sensor World
      mask Help:
      | Sends signal(s) from Simulink to the Sensor World.
      | 
      | - Port Name [-]: specifies the name of the output terminal of the Simulink block.
      | - Index [-]: specifies the start position in the output vector sent to the Sensor World
      | - Port dimensions [-]: specifies the width (number of scalars) of the output port
      | - Upload period [s]: specifies the upload period (in seconds) of the port.
      mask Display: port_label('input', 1, PortName)
  wires:
  CasingLights/1 -> Demux4/1
  Demux4/3 -> Saturation3/1
  Demux4/2 -> Saturation2/1
  Demux4/1 -> Saturation1/1
  Saturation1/1 -> conv_Red/1(on_off)
  Saturation2/1 -> conv_Orange/1(on_off)
  Saturation3/1 -> conv_Green/1(on_off)
  conv_Red/1(RGBcolor) -> visu_CasingRed/1(Y)
  conv_Orange/1(RGBcolor) -> visu_CasingOrange/1(Y)
  conv_Green/1(RGBcolor) -> visu_CasingGreen/1(Y)

== system MCity_cs_withAEBSBlock/VISUCasingLights_1_TrafficLightDoubleUS_6 ==
  CasingLights : Inport
  Demux4 : Demux  Outputs=3
  Saturation1 : Saturate  UpperLimit=1  LowerLimit=0
  Saturation2 : Saturate  UpperLimit=1  LowerLimit=0
  Saturation3 : Saturate  UpperLimit=1  LowerLimit=0
  conv_Green : Subsystem
  conv_Orange : Subsystem
  conv_Red : Subsystem
  visu_CasingGreen : Subsystem  mask(ToSensorWorld){PortName=visu_LightCasingGreen_1, PortIndex=414, PortWidth=16, TimeStep=1/200}
      mask prompts: PortName "Port Name [-]"; PortIndex "Index [-]"; PortWidth "Port Dimensions [-]"; TimeStep "Upload Period [s]"
      mask help: Sends signal(s) from Simulink to the Sensor World
      mask Help:
      | Sends signal(s) from Simulink to the Sensor World.
      | 
      | - Port Name [-]: specifies the name of the output terminal of the Simulink block.
      | - Index [-]: specifies the start position in the output vector sent to the Sensor World
      | - Port dimensions [-]: specifies the width (number of scalars) of the output port
      | - Upload period [s]: specifies the upload period (in seconds) of the port.
      mask Display: port_label('input', 1, PortName)
  visu_CasingOrange : Subsystem  mask(ToSensorWorld){PortName=visu_LightCasingOrange_1, PortIndex=430, PortWidth=16, TimeStep=1/200}
      mask prompts: PortName "Port Name [-]"; PortIndex "Index [-]"; PortWidth "Port Dimensions [-]"; TimeStep "Upload Period [s]"
      mask help: Sends signal(s) from Simulink to the Sensor World
      mask Help:
      | Sends signal(s) from Simulink to the Sensor World.
      | 
      | - Port Name [-]: specifies the name of the output terminal of the Simulink block.
      | - Index [-]: specifies the start position in the output vector sent to the Sensor World
      | - Port dimensions [-]: specifies the width (number of scalars) of the output port
      | - Upload period [s]: specifies the upload period (in seconds) of the port.
      mask Display: port_label('input', 1, PortName)
  visu_CasingRed : Subsystem  mask(ToSensorWorld){PortName=visu_LightCasingRed_1, PortIndex=446, PortWidth=16, TimeStep=1/200}
      mask prompts: PortName "Port Name [-]"; PortIndex "Index [-]"; PortWidth "Port Dimensions [-]"; TimeStep "Upload Period [s]"
      mask help: Sends signal(s) from Simulink to the Sensor World
      mask Help:
      | Sends signal(s) from Simulink to the Sensor World.
      | 
      | - Port Name [-]: specifies the name of the output terminal of the Simulink block.
      | - Index [-]: specifies the start position in the output vector sent to the Sensor World
      | - Port dimensions [-]: specifies the width (number of scalars) of the output port
      | - Upload period [s]: specifies the upload period (in seconds) of the port.
      mask Display: port_label('input', 1, PortName)
  wires:
  CasingLights/1 -> Demux4/1
  Demux4/3 -> Saturation3/1
  Demux4/2 -> Saturation2/1
  Demux4/1 -> Saturation1/1
  Saturation1/1 -> conv_Red/1(on_off)
  Saturation2/1 -> conv_Orange/1(on_off)
  Saturation3/1 -> conv_Green/1(on_off)
  conv_Red/1(RGBcolor) -> visu_CasingRed/1(Y)
  conv_Orange/1(RGBcolor) -> visu_CasingOrange/1(Y)
  conv_Green/1(RGBcolor) -> visu_CasingGreen/1(Y)

== system MCity_cs_withAEBSBlock/VISUCasingLights_1_TrafficLightDoubleUS_7 ==
  CasingLights : Inport
  Demux4 : Demux  Outputs=3
  Saturation1 : Saturate  UpperLimit=1  LowerLimit=0
  Saturation2 : Saturate  UpperLimit=1  LowerLimit=0
  Saturation3 : Saturate  UpperLimit=1  LowerLimit=0
  conv_Green : Subsystem
  conv_Orange : Subsystem
  conv_Red : Subsystem
  visu_CasingGreen : Subsystem  mask(ToSensorWorld){PortName=visu_LightCasingGreen_1, PortIndex=606, PortWidth=16, TimeStep=1/200}
      mask prompts: PortName "Port Name [-]"; PortIndex "Index [-]"; PortWidth "Port Dimensions [-]"; TimeStep "Upload Period [s]"
      mask help: Sends signal(s) from Simulink to the Sensor World
      mask Help:
      | Sends signal(s) from Simulink to the Sensor World.
      | 
      | - Port Name [-]: specifies the name of the output terminal of the Simulink block.
      | - Index [-]: specifies the start position in the output vector sent to the Sensor World
      | - Port dimensions [-]: specifies the width (number of scalars) of the output port
      | - Upload period [s]: specifies the upload period (in seconds) of the port.
      mask Display: port_label('input', 1, PortName)
  visu_CasingOrange : Subsystem  mask(ToSensorWorld){PortName=visu_LightCasingOrange_1, PortIndex=622, PortWidth=16, TimeStep=1/200}
      mask prompts: PortName "Port Name [-]"; PortIndex "Index [-]"; PortWidth "Port Dimensions [-]"; TimeStep "Upload Period [s]"
      mask help: Sends signal(s) from Simulink to the Sensor World
      mask Help:
      | Sends signal(s) from Simulink to the Sensor World.
      | 
      | - Port Name [-]: specifies the name of the output terminal of the Simulink block.
      | - Index [-]: specifies the start position in the output vector sent to the Sensor World
      | - Port dimensions [-]: specifies the width (number of scalars) of the output port
      | - Upload period [s]: specifies the upload period (in seconds) of the port.
      mask Display: port_label('input', 1, PortName)
  visu_CasingRed : Subsystem  mask(ToSensorWorld){PortName=visu_LightCasingRed_1, PortIndex=638, PortWidth=16, TimeStep=1/200}
      mask prompts: PortName "Port Name [-]"; PortIndex "Index [-]"; PortWidth "Port Dimensions [-]"; TimeStep "Upload Period [s]"
      mask help: Sends signal(s) from Simulink to the Sensor World
      mask Help:
      | Sends signal(s) from Simulink to the Sensor World.
      | 
      | - Port Name [-]: specifies the name of the output terminal of the Simulink block.
      | - Index [-]: specifies the start position in the output vector sent to the Sensor World
      | - Port dimensions [-]: specifies the width (number of scalars) of the output port
      | - Upload period [s]: specifies the upload period (in seconds) of the port.
      mask Display: port_label('input', 1, PortName)
  wires:
  CasingLights/1 -> Demux4/1
  Demux4/3 -> Saturation3/1
  Demux4/2 -> Saturation2/1
  Demux4/1 -> Saturation1/1
  Saturation1/1 -> conv_Red/1(on_off)
  Saturation2/1 -> conv_Orange/1(on_off)
  Saturation3/1 -> conv_Green/1(on_off)
  conv_Red/1(RGBcolor) -> visu_CasingRed/1(Y)
  conv_Orange/1(RGBcolor) -> visu_CasingOrange/1(Y)
  conv_Green/1(RGBcolor) -> visu_CasingGreen/1(Y)

== system MCity_cs_withAEBSBlock/VISUCasingLights_1_TrafficLightDoubleUS_8 ==
  CasingLights : Inport
  Demux4 : Demux  Outputs=3
  Saturation1 : Saturate  UpperLimit=1  LowerLimit=0
  Saturation2 : Saturate  UpperLimit=1  LowerLimit=0
  Saturation3 : Saturate  UpperLimit=1  LowerLimit=0
  conv_Green : Subsystem
  conv_Orange : Subsystem
  conv_Red : Subsystem
  visu_CasingGreen : Subsystem  mask(ToSensorWorld){PortName=visu_LightCasingGreen_1, PortIndex=990, PortWidth=16, TimeStep=1/200}
      mask prompts: PortName "Port Name [-]"; PortIndex "Index [-]"; PortWidth "Port Dimensions [-]"; TimeStep "Upload Period [s]"
      mask help: Sends signal(s) from Simulink to the Sensor World
      mask Help:
      | Sends signal(s) from Simulink to the Sensor World.
      | 
      | - Port Name [-]: specifies the name of the output terminal of the Simulink block.
      | - Index [-]: specifies the start position in the output vector sent to the Sensor World
      | - Port dimensions [-]: specifies the width (number of scalars) of the output port
      | - Upload period [s]: specifies the upload period (in seconds) of the port.
      mask Display: port_label('input', 1, PortName)
  visu_CasingOrange : Subsystem  mask(ToSensorWorld){PortName=visu_LightCasingOrange_1, PortIndex=1006, PortWidth=16, TimeStep=1/200}
      mask prompts: PortName "Port Name [-]"; PortIndex "Index [-]"; PortWidth "Port Dimensions [-]"; TimeStep "Upload Period [s]"
      mask help: Sends signal(s) from Simulink to the Sensor World
      mask Help:
      | Sends signal(s) from Simulink to the Sensor World.
      | 
      | - Port Name [-]: specifies the name of the output terminal of the Simulink block.
      | - Index [-]: specifies the start position in the output vector sent to the Sensor World
      | - Port dimensions [-]: specifies the width (number of scalars) of the output port
      | - Upload period [s]: specifies the upload period (in seconds) of the port.
      mask Display: port_label('input', 1, PortName)
  visu_CasingRed : Subsystem  mask(ToSensorWorld){PortName=visu_LightCasingRed_1, PortIndex=1022, PortWidth=16, TimeStep=1/200}
      mask prompts: PortName "Port Name [-]"; PortIndex "Index [-]"; PortWidth "Port Dimensions [-]"; TimeStep "Upload Period [s]"
      mask help: Sends signal(s) from Simulink to the Sensor World
      mask Help:
      | Sends signal(s) from Simulink to the Sensor World.
      | 
      | - Port Name [-]: specifies the name of the output terminal of the Simulink block.
      | - Index [-]: specifies the start position in the output vector sent to the Sensor World
      | - Port dimensions [-]: specifies the width (number of scalars) of the output port
      | - Upload period [s]: specifies the upload period (in seconds) of the port.
      mask Display: port_label('input', 1, PortName)
  wires:
  CasingLights/1 -> Demux4/1
  Demux4/3 -> Saturation3/1
  Demux4/2 -> Saturation2/1
  Demux4/1 -> Saturation1/1
  Saturation1/1 -> conv_Red/1(on_off)
  Saturation2/1 -> conv_Orange/1(on_off)
  Saturation3/1 -> conv_Green/1(on_off)
  conv_Red/1(RGBcolor) -> visu_CasingRed/1(Y)
  conv_Orange/1(RGBcolor) -> visu_CasingOrange/1(Y)
  conv_Green/1(RGBcolor) -> visu_CasingGreen/1(Y)
